simulink model "MotorControlSim_OpenLoopPWM"  (R2025b)
settings: Solver=FixedStepAuto  FixedStep=1e-6
libraries: slpidlib x2, simulink x1
(part 1 of 2)
settings Model: Creator=azmib
settings SolverCC: ZeroCrossControl=EnableAll  MaxZcPerStep=100.0
settings SimscapeCC: SimscapeNominalValues="[{\"value\":\"1\",\"unit\":\"A\"},{\"value\":\"1\",\"unit\":\"bar\"},{\"value\":\"1\",\"unit\":\"cm^2\"},{\"value\":\"1\",\"unit\":\"cm^3/s\"},{\"value\":\"1\",\"unit\":\"kJ/kg\"},{\"value\":\"1\",\"unit\":\"kW\"},{\"value\":\"1\",\"unit\":\"l\"},{\"value\":\"1\",\"unit\":\"N\"},{\"value\":\"1\",\"unit\":\"N*m\"},{\"value\":\"1\",\"unit\":\"V\"},{\"value\":\"0.001\",\"unit\":\"Wb\"}]"  SimscapeLogType=all  SimscapeLogDataHistory=10000.0

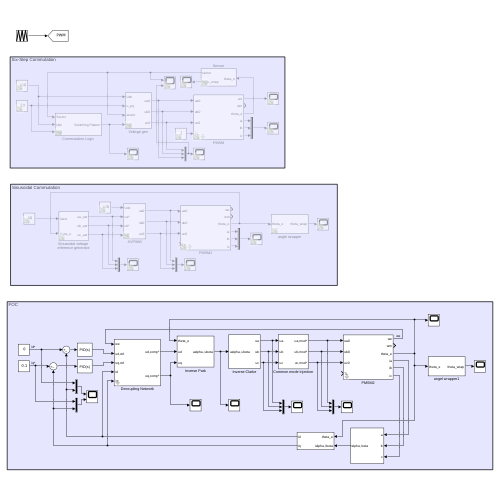
[thumbnail: Simulink's stored preview of the top-level diagram]
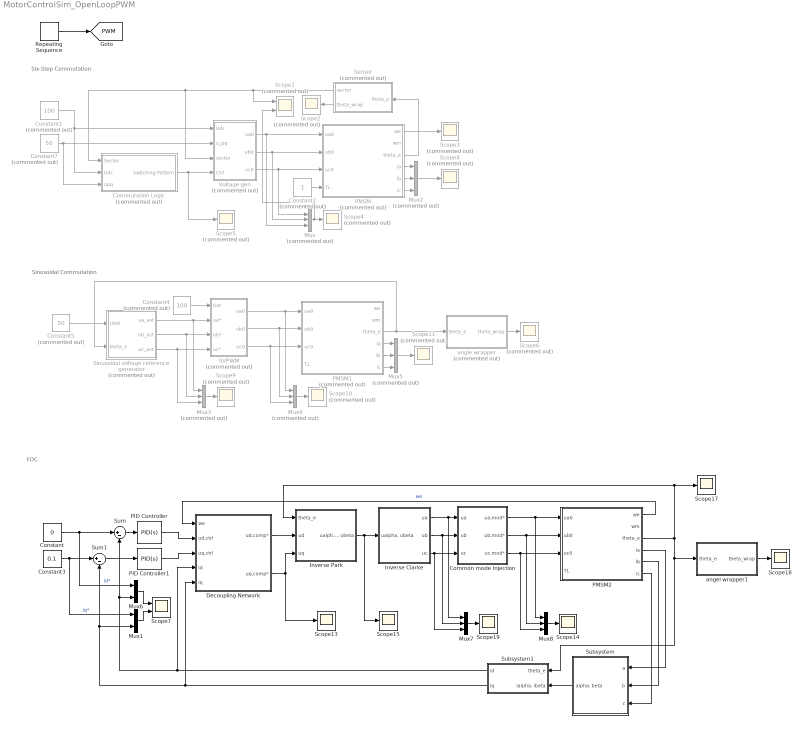
== system MotorControlSim_OpenLoopPWM ==
  note: FOC
  note: Sinusoidal Commutation
  note: Six-Step Commutation
  Common mode Injection : Subsystem
  Commutation Logic : Subsystem  Commented=on
  Constant : Constant  Value=0
  Constant1 : Constant  Commented=on  Value=100
  Constant2 : Constant  Commented=on
  Constant3 : Constant  Value=0.1
  Constant4 : Constant  Commented=on  Value=100
  Constant5 : Constant  Commented=on  Value=50
  Constant7 : Constant  Commented=on  Value=50
  Decoupling Network : Subsystem  mask{Ls=0.002, psi_PM=0.018}
      mask prompts: Ls "pq Inductance"; psi_PM "Permanent magnet flux"
  Inverse Clarke : Subsystem
  Inverse Park : Subsystem
  Mux{,2..5} (5 alike) : Mux  Commented=on  Inputs=3
  Mux1 : Mux  Inputs=2
  Mux6 : Mux  Inputs=2
  Mux7 : Mux  Inputs=3
  Mux8 : Mux  Inputs=3
  PID Controller : slpidlib/PID Controller  Controller=PID  Form=Parallel  TimeDomain=Continuous-time  UseExternalTs=off  SampleTime=-1  IntegratorMethod=Forward Euler  FilterMethod=Forward Euler  ControllerParametersSource=internal  P=15  I=250  UseKiTs=off  D=0  UseExternalDerivativeSource=off  N=100  UseFilter=on  TunerSelectOption=Transfer Function Based (PID Tuner App)  InitialConditionSource=internal  InitialConditionForIntegrator=0  InitialConditionForFilter=0  DifferentiatorICPrevScaledInput=0  ExternalReset=none  TrackingMode=off  Kt=1  LimitOutput=off  SatLimitsSource=internal  UpperSaturationLimit=inf  LowerSaturationLimit=-inf  LinearizeAsGain=on  AntiWindupMode=none  Kb=1  LimitIntegrator=off  UpperIntegratorSaturationLimit=inf  LowerIntegratorSaturationLimit=-inf  POutMin=[]  POutMax=[]  IOutMin=[]  IOutMax=[]  DOutMin=[]  DOutMax=[]  NOutMin=[]  NOutMax=[]  SumOutMin=[]  SumOutMax=[]  SaturationOutMin=[]  SaturationOutMax=[]  PParamMin=[]  PParamMax=[]  IParamMin=[]  IParamMax=[]  DParamMin=[]  DParamMax=[]  NParamMin=[]  NParamMax=[]  KbParamMin=[]  KbParamMax=[]  KtParamMin=[]  KtParamMax=[]  KbOutMin=[]  KbOutMax=[]  KtOutMin=[]  KtOutMax=[]  IntegratorOutMin=[]  IntegratorOutMax=[]  FilterOutMin=[]  FilterOutMax=[]  SumI1OutMin=[]  SumI1OutMax=[]  SumI2OutMin=[]  SumI2OutMax=[]  SumI3OutMin=[]  SumI3OutMax=[]  SumI4OutMin=[]  SumI4OutMax=[]  SumDOutMin=[]  SumDOutMax=[]  DifferentiatorOutMin=[]  DifferentiatorOutMax=[]  FilterDiffOutCoefMin=[]  FilterDiffOutCoefMax=[]  ReciprocalOutMin=[]  ReciprocalOutMax=[]  SumDenOutMin=[]  SumDenOutMax=[]  SumNumOutMin=[]  SumNumOutMax=[]  DivideOutMin=[]  DivideOutMax=[]  UdiffTsProdOutMin=[]  UdiffTsProdOutMax=[]  NTsProdOutMin=[]  NTsProdOutMax=[]  UintegralTsProdOutMin=[]  UintegralTsProdOutMax=[]  UngainTsProdOutMin=[]  UngainTsProdOutMax=[]  ClampingZeroOutDataTypeStr=Inherit: Inherit via back propagation  ClampingZeroOutMin=[]  ClampingZeroOutMax=[]  FilterDenConstantOutDataTypeStr=Inherit: Inherit via back propagation  FilterDenConstantOutMin=[]  FilterDenConstantOutMax=[]  PCopyOutDataTypeStr=Inherit: Inherit via back propagation  PCopyOutMin=[]  PCopyOutMax=[]  NCopyOutDataTypeStr=Inherit: Inherit via back propagation  NCopyOutMin=[]  NCopyOutMax=[]  IntegratorContinuousStateAttributes=''  IntegratorStateMustResolveToSignalObject=off  IntegratorRTWStateStorageClass=Auto  FilterContinuousStateAttributes=''  FilterStateMustResolveToSignalObject=off  FilterRTWStateStorageClass=Auto  ParallelPVariant=InternalParameters  IdealPVariant=Disabled  IVariant=InternalParameters  DVariant=InternalParameters  IntegratorVariant=Continuous  SatVariant=Disabled  AWVariant=Passthrough  PCopyVariant=Disabled  TRVariant=Disabled  FdbkBlocksVariant=Forward  IdealPFdbkVariant=Disabled  SatFdbkVariant=Disabled  DerivativeFilterVariant=ContFilter  NVariant=InternalParameters  NCopyVariant=Disabled  FilterICVariant=InternalICsFilter  IntegratorICVariant=InternalICs  ExternalResetVariant=Disabled  TRSumVariant=Passthrough  SumFdbkVariant=Disabled  SumVariant=Sum_PID  TsampFilterVariant=InternalTs  TsampNgainVariant=Passthrough  TsampIntegralVariant=Disabled_SignalSpec  ExternalSaturationOutDataTypeStr=Inherit: Same as second input  DerivativeSourceVariant=ErrorSignal  PreIntVariant=InternalPreInt
  PID Controller1 : slpidlib/PID Controller  Controller=PID  Form=Parallel  TimeDomain=Continuous-time  UseExternalTs=off  SampleTime=-1  IntegratorMethod=Forward Euler  FilterMethod=Forward Euler  ControllerParametersSource=internal  P=15  I=250  UseKiTs=off  D=0  UseExternalDerivativeSource=off  N=100  UseFilter=on  TunerSelectOption=Transfer Function Based (PID Tuner App)  InitialConditionSource=internal  InitialConditionForIntegrator=0  InitialConditionForFilter=0  DifferentiatorICPrevScaledInput=0  ExternalReset=none  TrackingMode=off  Kt=1  LimitOutput=off  SatLimitsSource=internal  UpperSaturationLimit=inf  LowerSaturationLimit=-inf  LinearizeAsGain=on  AntiWindupMode=none  Kb=1  LimitIntegrator=off  UpperIntegratorSaturationLimit=inf  LowerIntegratorSaturationLimit=-inf  POutMin=[]  POutMax=[]  IOutMin=[]  IOutMax=[]  DOutMin=[]  DOutMax=[]  NOutMin=[]  NOutMax=[]  SumOutMin=[]  SumOutMax=[]  SaturationOutMin=[]  SaturationOutMax=[]  PParamMin=[]  PParamMax=[]  IParamMin=[]  IParamMax=[]  DParamMin=[]  DParamMax=[]  NParamMin=[]  NParamMax=[]  KbParamMin=[]  KbParamMax=[]  KtParamMin=[]  KtParamMax=[]  KbOutMin=[]  KbOutMax=[]  KtOutMin=[]  KtOutMax=[]  IntegratorOutMin=[]  IntegratorOutMax=[]  FilterOutMin=[]  FilterOutMax=[]  SumI1OutMin=[]  SumI1OutMax=[]  SumI2OutMin=[]  SumI2OutMax=[]  SumI3OutMin=[]  SumI3OutMax=[]  SumI4OutMin=[]  SumI4OutMax=[]  SumDOutMin=[]  SumDOutMax=[]  DifferentiatorOutMin=[]  DifferentiatorOutMax=[]  FilterDiffOutCoefMin=[]  FilterDiffOutCoefMax=[]  ReciprocalOutMin=[]  ReciprocalOutMax=[]  SumDenOutMin=[]  SumDenOutMax=[]  SumNumOutMin=[]  SumNumOutMax=[]  DivideOutMin=[]  DivideOutMax=[]  UdiffTsProdOutMin=[]  UdiffTsProdOutMax=[]  NTsProdOutMin=[]  NTsProdOutMax=[]  UintegralTsProdOutMin=[]  UintegralTsProdOutMax=[]  UngainTsProdOutMin=[]  UngainTsProdOutMax=[]  ClampingZeroOutDataTypeStr=Inherit: Inherit via back propagation  ClampingZeroOutMin=[]  ClampingZeroOutMax=[]  FilterDenConstantOutDataTypeStr=Inherit: Inherit via back propagation  FilterDenConstantOutMin=[]  FilterDenConstantOutMax=[]  PCopyOutDataTypeStr=Inherit: Inherit via back propagation  PCopyOutMin=[]  PCopyOutMax=[]  NCopyOutDataTypeStr=Inherit: Inherit via back propagation  NCopyOutMin=[]  NCopyOutMax=[]  IntegratorContinuousStateAttributes=''  IntegratorStateMustResolveToSignalObject=off  IntegratorRTWStateStorageClass=Auto  FilterContinuousStateAttributes=''  FilterStateMustResolveToSignalObject=off  FilterRTWStateStorageClass=Auto  ParallelPVariant=InternalParameters  IdealPVariant=Disabled  IVariant=InternalParameters  DVariant=InternalParameters  IntegratorVariant=Continuous  SatVariant=Disabled  AWVariant=Passthrough  PCopyVariant=Disabled  TRVariant=Disabled  FdbkBlocksVariant=Forward  IdealPFdbkVariant=Disabled  SatFdbkVariant=Disabled  DerivativeFilterVariant=ContFilter  NVariant=InternalParameters  NCopyVariant=Disabled  FilterICVariant=InternalICsFilter  IntegratorICVariant=InternalICs  ExternalResetVariant=Disabled  TRSumVariant=Passthrough  SumFdbkVariant=Disabled  SumVariant=Sum_PID  TsampFilterVariant=InternalTs  TsampNgainVariant=Passthrough  TsampIntegralVariant=Disabled_SignalSpec  ExternalSaturationOutDataTypeStr=Inherit: Same as second input  DerivativeSourceVariant=ErrorSignal  PreIntVariant=InternalPreInt
  PMSM : Subsystem  Commented=on  mask(PMSM){Rs=0.045, Ls=0.002, psi_PM=0.018, p=14, J=2.5e-4, B=1e-3}
      mask prompts: Rs "Phase resistance [Rs]"; Ls "Direct- and  quadrature-axis inductances [Ls]"; psi_PM "Permanent magnet flux linkage [psi_PM]"; p "Pole pairs [p}"; J "Moment of inertia [J]"; B "viscous friction coefficient [B]"
      mask help: Mathematical model of a non-salient permanent magnet synchronous motor (PMSM).
  PMSM1 : Subsystem  Commented=on  mask(PMSM){Rs=0.045, Ls=0.002, psi_PM=0.018, p=14, J=2.5e-4, B=1e-3}
      mask prompts: Rs "Phase resistance [Rs]"; Ls "Direct- and  quadrature-axis inductances [Ls]"; psi_PM "Permanent magnet flux linkage [psi_PM]"; p "Pole pairs [p}"; J "Moment of inertia [J]"; B "viscous friction coefficient [B]"
      mask help: Mathematical model of a non-salient permanent magnet synchronous motor (PMSM).
  PMSM2 : Subsystem  mask(PMSM){Rs=0.045, Ls=0.002, psi_PM=0.018, p=14, J=2.5e-4, B=1e-3}
      mask prompts: Rs "Phase resistance [Rs]"; Ls "Direct- and  quadrature-axis inductances [Ls]"; psi_PM "Permanent magnet flux linkage [psi_PM]"; p "Pole pairs [p}"; J "Moment of inertia [J]"; B "viscous friction coefficient [B]"
      mask help: Mathematical model of a non-salient permanent magnet synchronous motor (PMSM).
  Repeating Sequence : simulink/Sources/Repeating Sequence  rep_seq_t=[0 0.00005 0.0001]  rep_seq_y=[0 1 0]
  SVPWM : Subsystem  Commented=on
  Scope1 : Scope  Commented=on  NumInputPorts=2
      settings: ActiveDisplayYMinimum=0.54492848630705648  ActiveDisplayYMaximum=6.21386272666987
  Scope{2..6,8..11} (9 alike) : Scope  Commented=on
      Scope10 settings: ActiveDisplayYMinimum=-12.499999999999996  ActiveDisplayYMaximum=112.5  DataLoggingVariableName=ScopeData10
      Scope11 settings: ActiveDisplayYMinimum=-61.952484857839465  ActiveDisplayYMaximum=66.897862739349023  DataLoggingVariableName=ScopeData11
      Scope2 settings: ActiveDisplayYMinimum=-44.997868385096346  ActiveDisplayYMaximum=404.99935148550094  DataLoggingVariableName=ScopeData2
      Scope3 settings: ActiveDisplayYMinimum=-84.895577173636241  ActiveDisplayYMaximum=93.106926628518693  DataLoggingVariableName=ScopeData3
      Scope4 settings: ActiveDisplayYMinimum=-12.499999999999996  ActiveDisplayYMaximum=112.5  DataLoggingVariableName=ScopeData4
      Scope5 settings: ActiveDisplayYMinimum=-0.14423076923076919  ActiveDisplayYMaximum=1.1057692307692308  DataLoggingVariableName=ScopeData5
      Scope6 settings: ActiveDisplayYMinimum=-556.861480878076  ActiveDisplayYMaximum=474.54651207001933  DataLoggingVariableName=ScopeData7
      Scope8 settings: ActiveDisplayYMinimum=-802.69476139838889  ActiveDisplayYMaximum=793.38425332468114  DataLoggingVariableName=ScopeData6
      Scope9 settings: ActiveDisplayYMinimum=-126.15384615374161  ActiveDisplayYMaximum=123.84615384570814  DataLoggingVariableName=ScopeData9
  Scope{13..15,17..19} (6 alike) : Scope
      Scope13 settings: ActiveDisplayYMinimum=-1.1385144753965966  ActiveDisplayYMaximum=7.7284276585384992  DataLoggingVariableName=ScopeData16
      Scope14 settings: ActiveDisplayYMinimum=-10.316497807088153  ActiveDisplayYMaximum=10.316497807088153  DataLoggingVariableName=ScopeData14
      Scope15 settings: ActiveDisplayYMinimum=-8.4790995533838753  ActiveDisplayYMaximum=8.4863578557596355  DataLoggingVariableName=ScopeData20
      Scope17 settings: ActiveDisplayYMinimum=-1061.0441841261031  ActiveDisplayYMaximum=9549.39765713493  DataLoggingVariableName=ScopeData17
      Scope18 settings: ActiveDisplayYMinimum=-449.98370924834887  ActiveDisplayYMaximum=449.99720138987811  DataLoggingVariableName=ScopeData18
      Scope19 settings: ActiveDisplayYMinimum=-11.80274291560826  ActiveDisplayYMaximum=11.802630733499404  DataLoggingVariableName=ScopeData19
  Scope7 : Scope  NumInputPorts=2
      settings: ActiveDisplayYMinimum=-5.6255188907389564E-5  ActiveDisplayYMaximum=0.0005062967001665062  DataLoggingVariableName=ScopeData13
  Sensor : Subsystem  Commented=on
  Sinusoidal voltage reference generator : Subsystem  Commented=on
  Subsystem : Subsystem
  Subsystem1 : Subsystem
  Sum : Sum  Inputs=|+-
  Sum1 : Sum  Inputs=|+-
  Voltage gen : Subsystem  Commented=on
  angel wrapper1 : Subsystem
  angle wrapper : Subsystem  Commented=on
  tag scope: PWM=global
  wires:
  Constant2/1 -> PMSM/4(TL)
  Sensor/1(sector) -> Voltage gen/3(sector), Commutation Logic/1(Sector), Scope1/1
  Commutation Logic/1(Switching Pattern) -> Scope5/1, Voltage gen/4(Ctrl)
  Voltage gen/2(ub0) -> Mux/2, PMSM/2(ub0)
  Voltage gen/1(ua0) -> Mux/3, PMSM/1(ua0)
  Voltage gen/3(uc0) -> Mux/1, PMSM/3(uc0)
  PMSM/3(theta_e) -> Sensor/1(theta_e)
  Sensor/2(theta_wrap) -> Scope2/1
  PMSM/1(we) -> Scope3/1
  Mux/1 -> Scope1/2, Scope4/1
  PMSM/5(ib) -> Mux2/2
  PMSM/4(ia) -> Mux2/1
  PMSM/6(ic) -> Mux2/3
  Mux2/1 -> Scope8/1
  PMSM1/3(theta_e) -> Sinusoidal voltage reference generator/2(theta_e), angle wrapper/1(theta_e)
  Sinusoidal voltage reference generator/1(ua_ast) -> Mux3/1, SVPWM/2(ua*)
  Sinusoidal voltage reference generator/2(ub_ast) -> Mux3/2, SVPWM/3(ub*)
  Sinusoidal voltage reference generator/3(uc_ast) -> Mux3/3, SVPWM/4(uc*)
  Mux3/1 -> Scope9/1
  SVPWM/1(ua0) -> PMSM1/1(ua0), Mux4/1
  SVPWM/2(ub0) -> PMSM1/2(ub0), Mux4/2
  SVPWM/3(uc0) -> PMSM1/3(uc0), Mux4/3
  Mux4/1 -> Scope10/1
  PMSM1/4(ia) -> Mux5/1
  PMSM1/5(ib) -> Mux5/2
  Mux5/1 -> Scope11/1
  PMSM1/6(ic) -> Mux5/3
  angle wrapper/1(theta_wrap) -> Scope6/1
  Mux7/1 -> Scope19/1
  Mux8/1 -> Scope14/1
  Inverse Clarke/2(ub) -> Mux7/2, Common mode Injection/2(ub)
  Inverse Clarke/1(ua) -> Mux7/1, Common mode Injection/1(ua)
  PMSM2/6(ic) -> Subsystem/3(c)
  PMSM2/3(theta_e) -> Subsystem1/1(theta_e), angel wrapper1/1(theta_e), Inverse Park/1(theta_e), Scope17/1
  angel wrapper1/1(theta_wrap) -> Scope18/1
  PMSM2/5(ib) -> Subsystem/2(b)
  PMSM2/4(ia) -> Subsystem/1(a)
  Inverse Clarke/3(uc) -> Mux7/3, Common mode Injection/3(uc)
  Inverse Park/1("ualpha, ubeta") -> Scope15/1, Inverse Clarke/1("ualpha, ubeta")
  Constant/1 -> Sum/1, Mux6/1  "id*"
  Constant3/1 -> Sum1/1, Mux1/1  "iq*"
  Decoupling Network/2(uq,comp*) -> Scope13/1, Inverse Park/3(uq)
  Decoupling Network/1(ud,comp*) -> Inverse Park/2(ud)
  PMSM2/1(we) -> Decoupling Network/1(we)  "we"
  Constant4/1 -> SVPWM/1(Udc)
  Constant5/1 -> Sinusoidal voltage reference generator/1(Uast)
  Mux1/1 -> Scope7/2
  Mux6/1 -> Scope7/1
  Constant1/1 -> Commutation Logic/2(Udc), Voltage gen/1(Udc)
  Constant7/1 -> Commutation Logic/3(upq), Voltage gen/2(u_pq)
  Common mode Injection/1(ua,mod*) -> Mux8/1, PMSM2/1(ua0)
  Common mode Injection/2(ub,mod*) -> Mux8/2, PMSM2/2(ub0)
  Common mode Injection/3(uc,mod*) -> Mux8/3, PMSM2/3(uc0)
  Repeating Sequence/1 -> [PWM]
  Subsystem/1("alpha, beta") -> Subsystem1/2("ialpha, ibeta")
  Subsystem1/1(id) -> Sum/2, Mux6/2, Decoupling Network/4(id)
  Subsystem1/2(iq) -> Sum1/2, Mux1/2, Decoupling Network/5(iq)
  Sum/1 -> PID Controller/1
  Sum1/1 -> PID Controller1/1
  PID Controller/1 -> Decoupling Network/2(ud,ctrl)
  PID Controller1/1 -> Decoupling Network/3(uq,ctrl)

== system MotorControlSim_OpenLoopPWM/Common mode Injection ==
  ua : Inport
  ub : Inport  Port=2
  uc : Inport  Port=3
  Add{,2..4} (4 alike) : Sum
  Gain : Gain  Gain=-1/2
  Max : MinMax  Function=max  Inputs=3
  Min : MinMax  Inputs=3
  ua,mod* : Outport
  ub,mod* : Outport  Port=2
  uc,mod* : Outport  Port=3
  wires:
  Add2/1 -> ua,mod*/1  "ua,mod*"
  Add3/1 -> ub,mod*/1  "ub,mod*"
  Min/1 -> Add/2
  Add4/1 -> uc,mod*/1  "uc,mod*"
  Add/1 -> Gain/1
  Gain/1 -> Add2/2, Add3/2, Add4/2  "u0"
  ub/1 -> Max/2, Min/2, Add3/1
  Max/1 -> Add/1
  uc/1 -> Max/3, Min/3, Add4/1
  ua/1 -> Min/1, Max/1, Add2/1

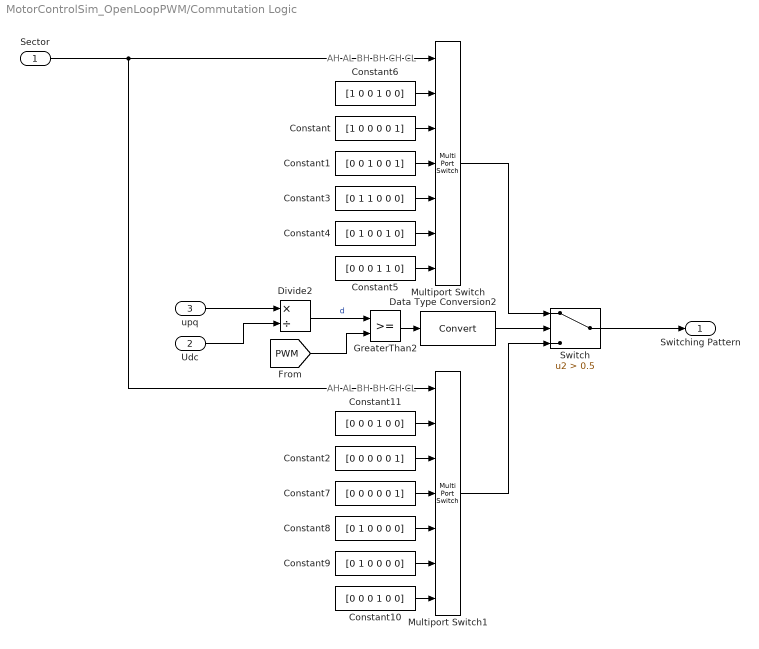
== system MotorControlSim_OpenLoopPWM/Commutation Logic ==
  note: AH AL BH BH CH CL
  note: AH AL BH BH CH CL
  Sector : Inport
  Udc : Inport  Port=2
  upq : Inport  Port=3
  Constant : Constant  Value=[1 0 0 0 0 1]
  Constant1 : Constant  Value=[0 0 1 0 0 1]
  Constant10 : Constant  Value=[0 0 0 1 0 0]
  Constant11 : Constant  Value=[0 0 0 1 0 0]
  Constant2 : Constant  Value=[0 0 0 0 0 1]
  Constant3 : Constant  Value=[0 1 1 0 0 0]
  Constant4 : Constant  Value=[0 1 0 0 1 0]
  Constant5 : Constant  Value=[0 0 0 1 1 0]
  Constant6 : Constant  Value=[1 0 0 1 0 0]
  Constant7 : Constant  Value=[0 0 0 0 0 1]
  Constant8 : Constant  Value=[0 1 0 0 0 0]
  Constant9 : Constant  Value=[0 1 0 0 0 0]
  Data Type Conversion2 : DataTypeConversion  SaturateOnIntegerOverflow=off  RndMeth=Floor
  Divide2 : Product  Inputs=*/
  GreaterThan2 : RelationalOperator  OutDataTypeStr=boolean  RndMeth=Simplest  InputSameDT=off
  Multiport Switch : MultiPortSwitch  Inputs=6  DiagnosticForDefault=None  SaturateOnIntegerOverflow=off  InputSameDT=off
  Multiport Switch1 : MultiPortSwitch  Inputs=6  DiagnosticForDefault=None  SaturateOnIntegerOverflow=off  InputSameDT=off
  Switch : Switch  Criteria=u2 > Threshold  Threshold=0.5  SaturateOnIntegerOverflow=off  InputSameDT=off
  Switching Pattern : Outport
  wires:
  Sector/1 -> Multiport Switch/1, Multiport Switch1/1
  Multiport Switch/1 -> Switch/1
  Multiport Switch1/1 -> Switch/3
  Switch/1 -> Switching Pattern/1
  Constant6/1 -> Multiport Switch/2
  Constant/1 -> Multiport Switch/3
  Constant1/1 -> Multiport Switch/4
  Constant3/1 -> Multiport Switch/5
  Constant5/1 -> Multiport Switch/7
  Constant4/1 -> Multiport Switch/6
  Constant11/1 -> Multiport Switch1/2
  Constant2/1 -> Multiport Switch1/3
  Constant7/1 -> Multiport Switch1/4
  Constant9/1 -> Multiport Switch1/6
  Constant10/1 -> Multiport Switch1/7
  Constant8/1 -> Multiport Switch1/5
  Udc/1 -> Divide2/2
  upq/1 -> Divide2/1
  [PWM] -> GreaterThan2/2
  GreaterThan2/1 -> Data Type Conversion2/1
  Divide2/1 -> GreaterThan2/1  "d"
  Data Type Conversion2/1 -> Switch/2

== system MotorControlSim_OpenLoopPWM/Decoupling Network ==
  we : Inport
  ud,ctrl : Inport  Port=2
  uq,ctrl : Inport  Port=3
  id : Inport  Port=4
  iq : Inport  Port=5
  Add : Sum
  Add4 : Sum  Inputs=+-
  Add5 : Sum
  Constant4 : Constant  Value=psi_PM
  Gain1 : Gain  Gain=Ls
  Gain2 : Gain  Gain=Ls
  Product : Product
  Product1 : Product
  ud,comp* : Outport
  uq,comp* : Outport  Port=2
  wires:
  iq/1 -> Product/1
  Product1/1 -> Add4/2
  Add5/1 -> Product1/2
  Constant4/1 -> Add5/2
  Gain2/1 -> Add5/1
  Add4/1 -> uq,comp*/1  "ud,comp*"
  Product/1 -> Gain1/1
  Gain1/1 -> Add/2
  ud,ctrl/1 -> Add/1
  id/1 -> Gain2/1
  Add/1 -> ud,comp*/1  "ud,comp*"
  we/1 -> Product1/1, Product/2
  uq,ctrl/1 -> Add4/1

== system MotorControlSim_OpenLoopPWM/Inverse Clarke ==
  "ualpha, ubeta" : Inport
  Constant1 : Constant  Value=[1 0; -1/2 sqrt(3)/2; -1/2 -sqrt(3)/2]
  Demux1 : Demux  Outputs=3
  Matrix Multiply : Product  Multiplication=Matrix(*)
  ua : Outport
  ub : Outport  Port=2
  uc : Outport  Port=3
  wires:
  Matrix Multiply/1 -> Demux1/1
  Constant1/1 -> Matrix Multiply/1
  Demux1/2 -> ub/1
  Demux1/3 -> uc/1
  Demux1/1 -> ua/1
  "ualpha, ubeta"/1 -> Matrix Multiply/2

== system MotorControlSim_OpenLoopPWM/Inverse Park ==
  theta_e : Inport
  ud : Inport  Port=2
  uq : Inport  Port=3
  Cos : Trigonometry  Operator=cos
  Gain3 : Gain  Gain=-1
  Matrix Concatenate3 : Concatenate  Mode=Multidimensional array  ConcatenateDimension=2
  Matrix Concatenate4 : Concatenate  Mode=Multidimensional array  ConcatenateDimension=2
  Matrix Concatenate5 : Concatenate  Mode=Multidimensional array
  Mux1 : Mux  Inputs=2
  Product2 : Product  Multiplication=Matrix(*)
  Sin2 : Trigonometry
  "ualpha, ubeta" : Outport
  wires:
  theta_e/1 -> Sin2/1, Cos/1
  Gain3/1 -> Matrix Concatenate3/2
  Cos/1 -> Matrix Concatenate3/1, Matrix Concatenate4/2
  Mux1/1 -> Product2/2
  uq/1 -> Mux1/2
  Matrix Concatenate4/1 -> Matrix Concatenate5/2
  Matrix Concatenate5/1 -> Product2/1
  Product2/1 -> "ualpha, ubeta"/1
  Sin2/1 -> Matrix Concatenate4/1, Gain3/1
  Matrix Concatenate3/1 -> Matrix Concatenate5/1
  ud/1 -> Mux1/1

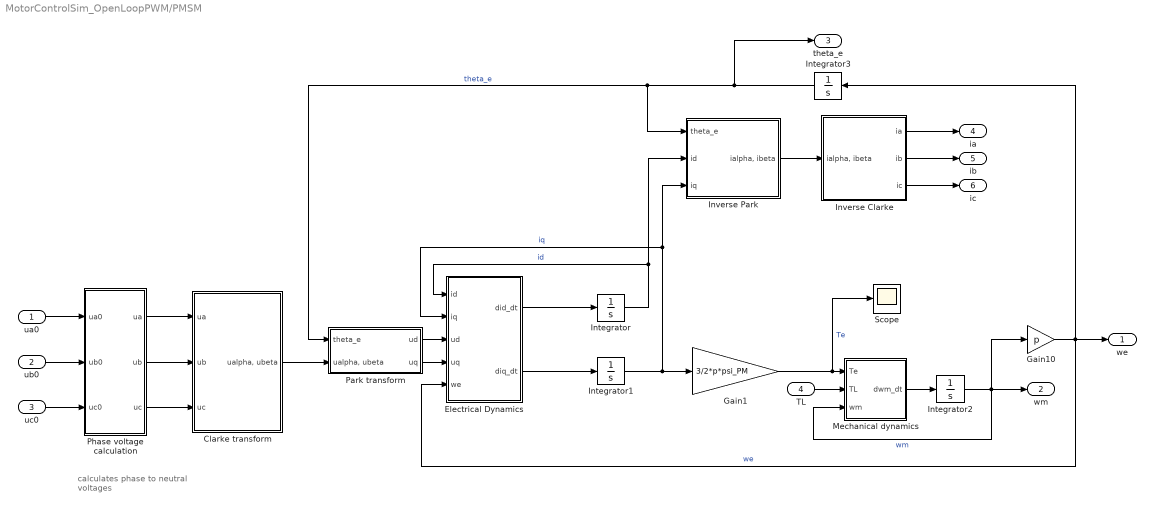
== system MotorControlSim_OpenLoopPWM/PMSM ==
  note: calculates phase to
      | neutral voltages
  ua0 : Inport  Unit=V
  ub0 : Inport  Port=2  Unit=V
  uc0 : Inport  Port=3  Unit=V
  TL : Inport  Port=4
  Clarke transform : Subsystem
  Electrical Dynamics : Subsystem
  Gain1 : Gain  Gain=3/2*p*psi_PM
  Gain10 : Gain  Gain=p
  Integrator{,1..3} (4 alike) : Integrator
  Inverse Clarke : Subsystem
  Inverse Park : Subsystem
  Mechanical dynamics : Subsystem
  Park transform : Subsystem
  Phase voltage calculation : Subsystem
  Scope : Scope
      settings: ActiveDisplayYMinimum=0.88625844411927557  ActiveDisplayYMaximum=1.0374557261199451
  we : Outport
  wm : Outport  Port=2
  theta_e : Outport  Port=3
  ia : Outport  Port=4
  ib : Outport  Port=5
  ic : Outport  Port=6
  wires:
  Integrator3/1 -> Park transform/1(theta_e), Inverse Park/1(theta_e), theta_e/1  "theta_e"
  Gain10/1 -> Integrator3/1, Electrical Dynamics/5(we), we/1  "we"
  Integrator1/1 -> Electrical Dynamics/2(iq), Inverse Park/3(iq), Gain1/1  "iq"
  Gain1/1 -> Scope/1, Mechanical dynamics/1(Te)  "Te"
  TL/1 -> Mechanical dynamics/2(TL)
  Mechanical dynamics/1(dwm_dt) -> Integrator2/1
  Integrator2/1 -> Mechanical dynamics/3(wm), Gain10/1, wm/1  "wm"
  Integrator/1 -> Electrical Dynamics/1(id), Inverse Park/2(id)  "id"
  Electrical Dynamics/1(did_dt) -> Integrator/1
  Electrical Dynamics/2(diq_dt) -> Integrator1/1
  Inverse Park/1("ialpha, ibeta") -> Inverse Clarke/1("ialpha, ibeta")
  Inverse Clarke/2(ib) -> ib/1
  Inverse Clarke/1(ia) -> ia/1
  Inverse Clarke/3(ic) -> ic/1
  Clarke transform/1("ualpha, ubeta") -> Park transform/2("ualpha, ubeta")
  Park transform/1(ud) -> Electrical Dynamics/3(ud)
  Park transform/2(uq) -> Electrical Dynamics/4(uq)
  ub0/1 -> Phase voltage calculation/2(ub0)
  ua0/1 -> Phase voltage calculation/1(ua0)
  uc0/1 -> Phase voltage calculation/3(uc0)
  Phase voltage calculation/2(ub) -> Clarke transform/2(ub)
  Phase voltage calculation/1(ua) -> Clarke transform/1(ua)
  Phase voltage calculation/3(uc) -> Clarke transform/3(uc)

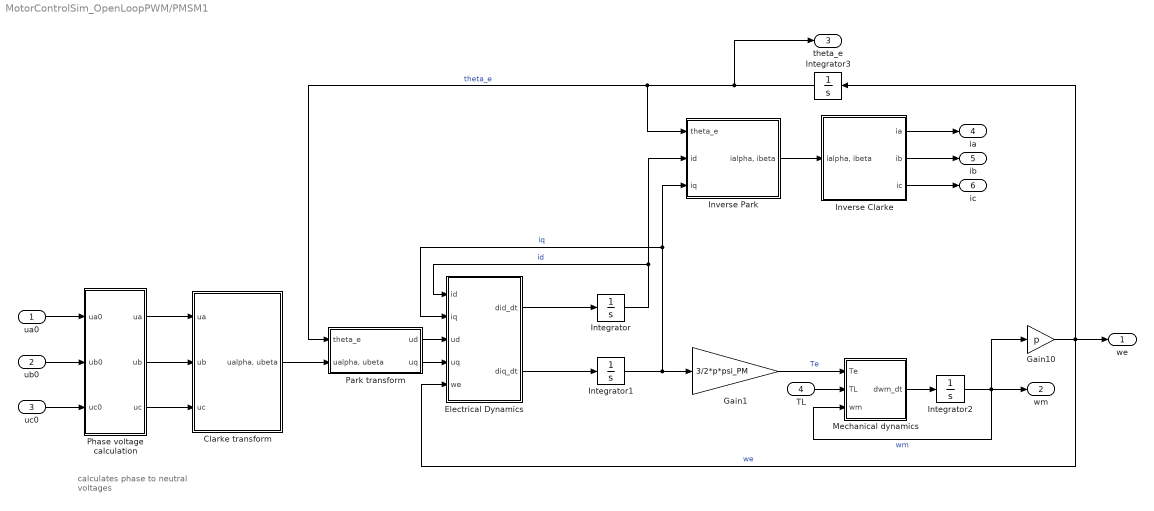
== system MotorControlSim_OpenLoopPWM/PMSM1 ==
  note: calculates phase to
      | neutral voltages
  ua0 : Inport  Unit=V
  ub0 : Inport  Port=2  Unit=V
  uc0 : Inport  Port=3  Unit=V
  TL : Inport  Port=4
  Clarke transform : Subsystem
  Electrical Dynamics : Subsystem
  Gain1 : Gain  Gain=3/2*p*psi_PM
  Gain10 : Gain  Gain=p
  Integrator{,1..3} (4 alike) : Integrator
  Inverse Clarke : Subsystem
  Inverse Park : Subsystem
  Mechanical dynamics : Subsystem
  Park transform : Subsystem
  Phase voltage calculation : Subsystem
  we : Outport
  wm : Outport  Port=2
  theta_e : Outport  Port=3
  ia : Outport  Port=4
  ib : Outport  Port=5
  ic : Outport  Port=6
  wires:
  Integrator3/1 -> Park transform/1(theta_e), Inverse Park/1(theta_e), theta_e/1  "theta_e"
  Gain10/1 -> Integrator3/1, Electrical Dynamics/5(we), we/1  "we"
  Integrator1/1 -> Electrical Dynamics/2(iq), Inverse Park/3(iq), Gain1/1  "iq"
  Gain1/1 -> Mechanical dynamics/1(Te)  "Te"
  TL/1 -> Mechanical dynamics/2(TL)
  Mechanical dynamics/1(dwm_dt) -> Integrator2/1
  Integrator2/1 -> Mechanical dynamics/3(wm), Gain10/1, wm/1  "wm"
  Integrator/1 -> Electrical Dynamics/1(id), Inverse Park/2(id)  "id"
  Electrical Dynamics/1(did_dt) -> Integrator/1
  Electrical Dynamics/2(diq_dt) -> Integrator1/1
  Inverse Park/1("ialpha, ibeta") -> Inverse Clarke/1("ialpha, ibeta")
  Inverse Clarke/2(ib) -> ib/1
  Inverse Clarke/1(ia) -> ia/1
  Inverse Clarke/3(ic) -> ic/1
  Clarke transform/1("ualpha, ubeta") -> Park transform/2("ualpha, ubeta")
  Park transform/1(ud) -> Electrical Dynamics/3(ud)
  Park transform/2(uq) -> Electrical Dynamics/4(uq)
  ub0/1 -> Phase voltage calculation/2(ub0)
  ua0/1 -> Phase voltage calculation/1(ua0)
  uc0/1 -> Phase voltage calculation/3(uc0)
  Phase voltage calculation/2(ub) -> Clarke transform/2(ub)
  Phase voltage calculation/1(ua) -> Clarke transform/1(ua)
  Phase voltage calculation/3(uc) -> Clarke transform/3(uc)

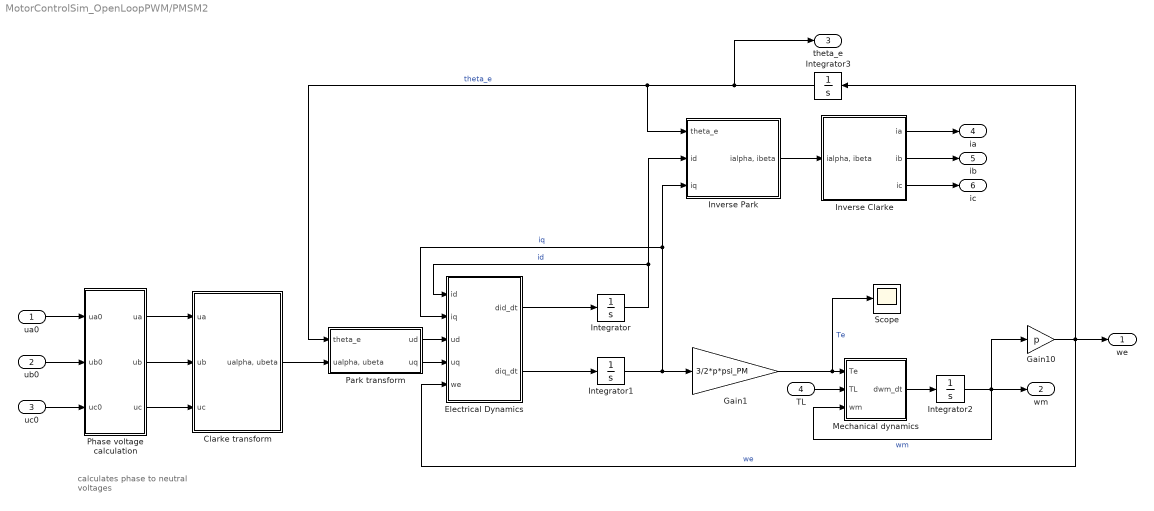
== system MotorControlSim_OpenLoopPWM/PMSM2 ==
  note: calculates phase to
      | neutral voltages
  ua0 : Inport  Unit=V
  ub0 : Inport  Port=2  Unit=V
  uc0 : Inport  Port=3  Unit=V
  TL : Inport  Port=4
  Clarke transform : Subsystem
  Electrical Dynamics : Subsystem
  Gain1 : Gain  Gain=3/2*p*psi_PM
  Gain10 : Gain  Gain=p
  Integrator{,1..3} (4 alike) : Integrator
  Inverse Clarke : Subsystem
  Inverse Park : Subsystem
  Mechanical dynamics : Subsystem
  Park transform : Subsystem
  Phase voltage calculation : Subsystem
  Scope : Scope
      settings: ActiveDisplayYMinimum=0.88625844411927557  ActiveDisplayYMaximum=1.0374557261199451
  we : Outport
  wm : Outport  Port=2
  theta_e : Outport  Port=3
  ia : Outport  Port=4
  ib : Outport  Port=5
  ic : Outport  Port=6
  wires:
  Integrator3/1 -> Park transform/1(theta_e), Inverse Park/1(theta_e), theta_e/1  "theta_e"
  Gain10/1 -> Integrator3/1, Electrical Dynamics/5(we), we/1  "we"
  Integrator1/1 -> Electrical Dynamics/2(iq), Inverse Park/3(iq), Gain1/1  "iq"
  Gain1/1 -> Scope/1, Mechanical dynamics/1(Te)  "Te"
  TL/1 -> Mechanical dynamics/2(TL)
  Mechanical dynamics/1(dwm_dt) -> Integrator2/1
  Integrator2/1 -> Mechanical dynamics/3(wm), Gain10/1, wm/1  "wm"
  Integrator/1 -> Electrical Dynamics/1(id), Inverse Park/2(id)  "id"
  Electrical Dynamics/1(did_dt) -> Integrator/1
  Electrical Dynamics/2(diq_dt) -> Integrator1/1
  Inverse Park/1("ialpha, ibeta") -> Inverse Clarke/1("ialpha, ibeta")
  Inverse Clarke/2(ib) -> ib/1
  Inverse Clarke/1(ia) -> ia/1
  Inverse Clarke/3(ic) -> ic/1
  Clarke transform/1("ualpha, ubeta") -> Park transform/2("ualpha, ubeta")
  Park transform/1(ud) -> Electrical Dynamics/3(ud)
  Park transform/2(uq) -> Electrical Dynamics/4(uq)
  ub0/1 -> Phase voltage calculation/2(ub0)
  ua0/1 -> Phase voltage calculation/1(ua0)
  uc0/1 -> Phase voltage calculation/3(uc0)
  Phase voltage calculation/2(ub) -> Clarke transform/2(ub)
  Phase voltage calculation/1(ua) -> Clarke transform/1(ua)
  Phase voltage calculation/3(uc) -> Clarke transform/3(uc)

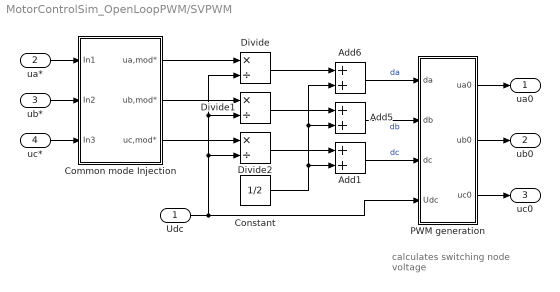
== system MotorControlSim_OpenLoopPWM/SVPWM ==
  note: calculates switching node
      | voltage
  Udc : Inport
  ua* : Inport  Port=2
  ub* : Inport  Port=3
  uc* : Inport  Port=4
  Add1 : Sum
  Add5 : Sum
  Add6 : Sum
  Common mode Injection : Subsystem
  Constant : Constant  Value=1/2
  Divide : Product  Inputs=*/
  Divide1 : Product  Inputs=*/
  Divide2 : Product  Inputs=*/
  PWM generation : Subsystem
  ua0 : Outport
  ub0 : Outport  Port=2
  uc0 : Outport  Port=3
  wires:
  Divide/1 -> Add6/1
  Divide1/1 -> Add5/1
  Divide2/1 -> Add1/1
  Constant/1 -> Add1/2, Add5/2, Add6/2
  Udc/1 -> PWM generation/4(Udc), Divide2/2, Divide1/2, Divide/2
  ua*/1 -> Common mode Injection/1(In1)
  ub*/1 -> Common mode Injection/2(In2)
  uc*/1 -> Common mode Injection/3(In3)
  Common mode Injection/1(ua,mod*) -> Divide/1
  Common mode Injection/2(ub,mod*) -> Divide1/1
  Common mode Injection/3(uc,mod*) -> Divide2/1
  Add6/1 -> PWM generation/1(da)  "da"
  Add5/1 -> PWM generation/2(db)  "db"
  Add1/1 -> PWM generation/3(dc)  "dc"
  PWM generation/1(ua0) -> ua0/1
  PWM generation/2(ub0) -> ub0/1
  PWM generation/3(uc0) -> uc0/1

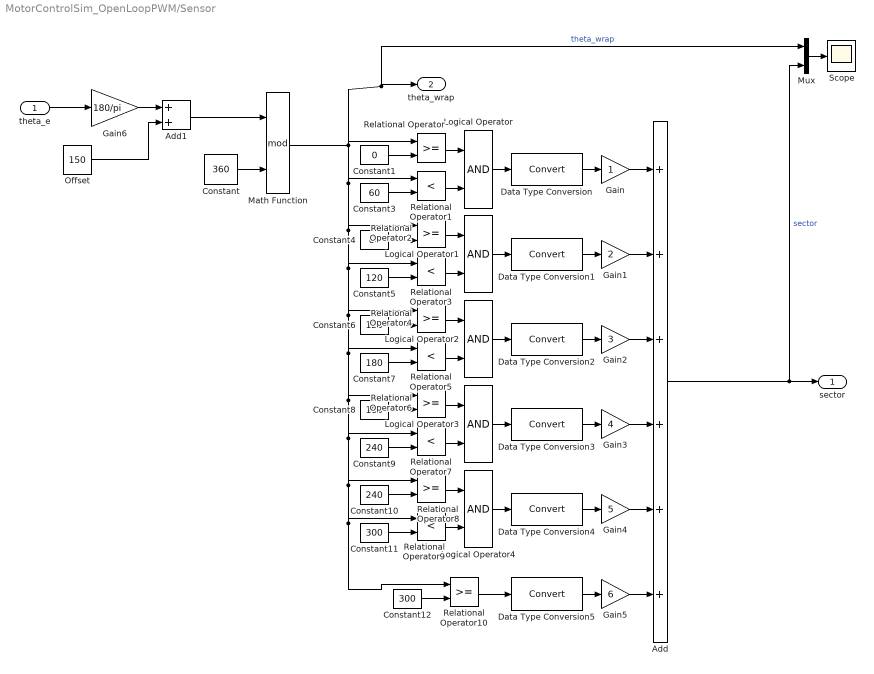
== system MotorControlSim_OpenLoopPWM/Sensor ==
  theta_e : Inport
  Add : Sum  Inputs=++++++
  Add1 : Sum
  Constant : Constant  Value=360
  Constant1 : Constant  Value=0
  Constant10 : Constant  Value=240
  Constant11 : Constant  Value=300
  Constant12 : Constant  Value=300
  Constant3 : Constant  Value=60
  Constant4 : Constant  Value=60
  Constant5 : Constant  Value=120
  Constant6 : Constant  Value=120
  Constant7 : Constant  Value=180
  Constant8 : Constant  Value=180
  Constant9 : Constant  Value=240
  Data Type Conversion{,1..5} (6 alike) : DataTypeConversion  SaturateOnIntegerOverflow=off  RndMeth=Floor
  Gain : Gain
  Gain1 : Gain  Gain=2
  Gain2 : Gain  Gain=3
  Gain3 : Gain  Gain=4
  Gain4 : Gain  Gain=5
  Gain5 : Gain  Gain=6
  Gain6 : Gain  Gain=180/pi
  Logical Operator{,1..4} (5 alike) : Logic  AllPortsSameDT=off  OutDataTypeStr=boolean
  Math Function : Math  Operator=mod
  Mux : Mux  Inputs=2
  Offset : Constant  Value=150
  Relational Operator{,2,4,6,8,10} (6 alike) : RelationalOperator  OutDataTypeStr=boolean  RndMeth=Simplest  InputSameDT=off
  Relational Operator{1,3,5,7,9} (5 alike) : RelationalOperator  Operator=<  OutDataTypeStr=boolean  RndMeth=Simplest  InputSameDT=off
  Scope : Scope
      settings: ActiveDisplayYMinimum=-39.26586921535646  ActiveDisplayYMaximum=393.39282293820821  DataLoggingVariableName=ScopeData8
  sector : Outport
  theta_wrap : Outport  Port=2
  wires:
  Data Type Conversion2/1 -> Gain2/1
  Constant5/1 -> Relational Operator3/2
  Relational Operator6/1 -> Logical Operator3/1
  Gain5/1 -> Add/6
  Gain3/1 -> Add/4
  Data Type Conversion5/1 -> Gain5/1
  Relational Operator7/1 -> Logical Operator3/2
  Gain2/1 -> Add/3
  Constant10/1 -> Relational Operator8/2
  Relational Operator4/1 -> Logical Operator2/1
  Constant/1 -> Math Function/2
  Constant8/1 -> Relational Operator6/2
  Math Function/1 -> Mux/1, theta_wrap/1, Relational Operator/1, Relational Operator2/1, Relational Operator4/1, Relational Operator10/1, Relational Operator9/1, Relational Operator8/1, Relational Operator7/1, Relational Operator6/1, Relational Operator5/1, Relational Operator3/1, Relational Operator1/1  "theta_wrap"
  Constant12/1 -> Relational Operator10/2
  Constant6/1 -> Relational Operator4/2
  Relational Operator2/1 -> Logical Operator1/1
  Logical Operator2/1 -> Data Type Conversion2/1
  Data Type Conversion1/1 -> Gain1/1
  Relational Operator1/1 -> Logical Operator/2
  Constant11/1 -> Relational Operator9/2
  Add/1 -> Mux/2, sector/1  "sector"
  Logical Operator3/1 -> Data Type Conversion3/1
  Relational Operator5/1 -> Logical Operator2/2
  Relational Operator/1 -> Logical Operator/1
  Gain4/1 -> Add/5
  Logical Operator/1 -> Data Type Conversion/1
  Data Type Conversion3/1 -> Gain3/1
  Gain/1 -> Add/1
  Constant7/1 -> Relational Operator5/2
  Constant3/1 -> Relational Operator1/2
  Relational Operator9/1 -> Logical Operator4/2
  Constant9/1 -> Relational Operator7/2
  Constant4/1 -> Relational Operator2/2
  Logical Operator1/1 -> Data Type Conversion1/1
  Data Type Conversion4/1 -> Gain4/1
  Constant1/1 -> Relational Operator/2
  Logical Operator4/1 -> Data Type Conversion4/1
  Data Type Conversion/1 -> Gain/1
  Gain1/1 -> Add/2
  Relational Operator3/1 -> Logical Operator1/2
  Relational Operator8/1 -> Logical Operator4/1
  theta_e/1 -> Gain6/1
  Relational Operator10/1 -> Data Type Conversion5/1
  Gain6/1 -> Add1/1
  Add1/1 -> Math Function/1
  Offset/1 -> Add1/2
  Mux/1 -> Scope/1

== system MotorControlSim_OpenLoopPWM/Sinusoidal voltage reference generator ==
  Uast : Inport
  theta_e : Inport  Port=2
  Constant : Constant  Value=2*pi/3
  Product : Product
  Product1 : Product
  Product2 : Product
  Sin : Trigonometry
  Sin1 : Trigonometry
  Sin2 : Trigonometry
  Sum1 : Sum  Inputs=|+-
  Sum2 : Sum  Inputs=|++
  ua_ast : Outport
  ub_ast : Outport  Port=2
  uc_ast : Outport  Port=3
  wires:
  Sum2/1 -> Sin2/1
  Product/1 -> uc_ast/1  "uc_ast"
  Sin1/1 -> Product1/2
  Constant/1 -> Sum2/2, Sum1/2
  Sum1/1 -> Sin1/1
  theta_e/1 -> Sin/1, Sum1/1, Sum2/1
  Sin2/1 -> Product/2
  Sin/1 -> Product2/2
  Product2/1 -> ua_ast/1  "ua_ast"
  Product1/1 -> ub_ast/1  "ub_ast"
  Uast/1 -> Product2/1, Product1/1, Product/1

== system MotorControlSim_OpenLoopPWM/Subsystem ==
  a : Inport
  b : Inport  Port=2
  c : Inport  Port=3
  Constant : Constant  Value=[1 -1/2 -1/2; 0 sqrt(3)/2 -sqrt(3)/2]
  Gain2 : Gain  Gain=2/3
  Mux : Mux  Inputs=3
  Product : Product  Multiplication=Matrix(*)
  "alpha, beta" : Outport
  wires:
  Gain2/1 -> Product/1
  b/1 -> Mux/2
  Constant/1 -> Gain2/1
  Mux/1 -> Product/2
  Product/1 -> "alpha, beta"/1
  c/1 -> Mux/3
  a/1 -> Mux/1

== system MotorControlSim_OpenLoopPWM/Subsystem1 ==
  theta_e : Inport
  "ialpha, ibeta" : Inport  Port=2
  Demux : Demux  Outputs=2
  Gain : Gain  Gain=-1
  Matrix Concatenate : Concatenate  Mode=Multidimensional array  ConcatenateDimension=2
  Matrix Concatenate1 : Concatenate  Mode=Multidimensional array  ConcatenateDimension=2
  Matrix Concatenate2 : Concatenate  Mode=Multidimensional array
  Product1 : Product  Multiplication=Matrix(*)
  Sin : Trigonometry  Operator=cos
  Sin1 : Trigonometry
  id : Outport
  iq : Outport  Port=2
  wires:
  Demux/2 -> iq/1  "uq"
  Product1/1 -> Demux/1  "ud, uq"
  Gain/1 -> Matrix Concatenate1/1
  Matrix Concatenate1/1 -> Matrix Concatenate2/2
  Sin1/1 -> Gain/1, Matrix Concatenate/2
  Matrix Concatenate2/1 -> Product1/1
  Matrix Concatenate/1 -> Matrix Concatenate2/1
  Sin/1 -> Matrix Concatenate/1, Matrix Concatenate1/2
  theta_e/1 -> Sin1/1, Sin/1
  Demux/1 -> id/1  "ud"
  "ialpha, ibeta"/1 -> Product1/2

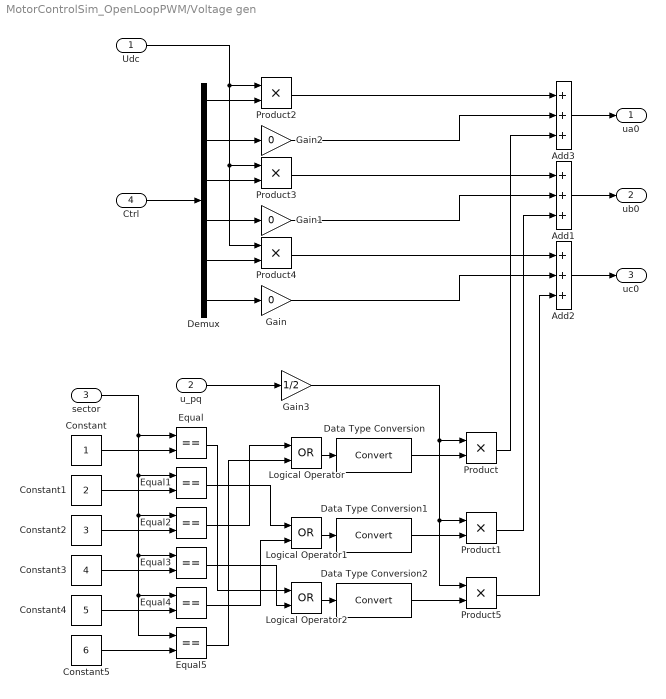
== system MotorControlSim_OpenLoopPWM/Voltage gen ==
  Udc : Inport
  u_pq : Inport  Port=2
  sector : Inport  Port=3
  Ctrl : Inport  Port=4
  Add1 : Sum  Inputs=+++
  Add2 : Sum  Inputs=+++
  Add3 : Sum  Inputs=+++
  Constant : Constant
  Constant1 : Constant  Value=2
  Constant2 : Constant  Value=3
  Constant3 : Constant  Value=4
  Constant4 : Constant  Value=5
  Constant5 : Constant  Value=6
  Data Type Conversion : DataTypeConversion  SaturateOnIntegerOverflow=off  RndMeth=Floor
  Data Type Conversion1 : DataTypeConversion  SaturateOnIntegerOverflow=off  RndMeth=Floor
  Data Type Conversion2 : DataTypeConversion  SaturateOnIntegerOverflow=off  RndMeth=Floor
  Demux : Demux  Outputs=6
  Equal{,1..5} (6 alike) : RelationalOperator  Operator===  OutDataTypeStr=boolean  RndMeth=Simplest  InputSameDT=off
  Gain : Gain  Gain=0
  Gain1 : Gain  Gain=0
  Gain2 : Gain  Gain=0
  Gain3 : Gain  Gain=1/2
  Logical Operator : Logic  Operator=OR  AllPortsSameDT=off  OutDataTypeStr=boolean
  Logical Operator1 : Logic  Operator=OR  AllPortsSameDT=off  OutDataTypeStr=boolean
  Logical Operator2 : Logic  Operator=OR  AllPortsSameDT=off  OutDataTypeStr=boolean
  Product{,1..5} (6 alike) : Product
  ua0 : Outport
  ub0 : Outport  Port=2
  uc0 : Outport  Port=3
  wires:
  Demux/3 -> Product3/2
  Udc/1 -> Product4/1, Product3/1, Product2/1
  Ctrl/1 -> Demux/1
  Demux/1 -> Product2/2
  Demux/5 -> Product4/2
  Product2/1 -> Add3/1
  Demux/6 -> Gain/1
  Demux/4 -> Gain1/1
  Demux/2 -> Gain2/1
  Gain2/1 -> Add3/2
  Data Type Conversion/1 -> Product/2
  Data Type Conversion1/1 -> Product1/2
  Data Type Conversion2/1 -> Product5/2
  Gain3/1 -> Product/1, Product1/1, Product5/1
  Product3/1 -> Add1/1
  Gain1/1 -> Add1/2
  Product4/1 -> Add2/1
  Gain/1 -> Add2/2
  Product/1 -> Add3/3
  Product1/1 -> Add1/3
  Product5/1 -> Add2/3
  Add3/1 -> ua0/1
  Add1/1 -> ub0/1
  Add2/1 -> uc0/1
  sector/1 -> Equal5/1, Equal4/1, Equal3/1, Equal2/1, Equal1/1, Equal/1
  Constant/1 -> Equal/2
  Constant1/1 -> Equal1/2
  Constant2/1 -> Equal2/2
  Constant3/1 -> Equal3/2
  Constant4/1 -> Equal4/2
  Constant5/1 -> Equal5/2
  Logical Operator/1 -> Data Type Conversion/1
  Logical Operator1/1 -> Data Type Conversion1/1
  Logical Operator2/1 -> Data Type Conversion2/1
  Equal2/1 -> Logical Operator/1
  Equal5/1 -> Logical Operator/2
  Equal1/1 -> Logical Operator1/1
  Equal4/1 -> Logical Operator1/2
  Equal3/1 -> Logical Operator2/2
  Equal/1 -> Logical Operator2/1
  u_pq/1 -> Gain3/1

== system MotorControlSim_OpenLoopPWM/angel wrapper1 ==
  theta_e : Inport
  Constant : Constant  Value=360
  Gain6 : Gain  Gain=180/pi
  Math Function : Math  Operator=rem
  theta_wrap : Outport
  wires:
  Constant/1 -> Math Function/2
  Gain6/1 -> Math Function/1  "theta_deg"
  theta_e/1 -> Gain6/1
  Math Function/1 -> theta_wrap/1  "theta_wrap"

== system MotorControlSim_OpenLoopPWM/angle wrapper ==
  theta_e : Inport
  Constant : Constant  Value=360
  Gain6 : Gain  Gain=180/pi
  Math Function : Math  Operator=rem
  theta_wrap : Outport
  wires:
  Constant/1 -> Math Function/2
  Gain6/1 -> Math Function/1  "theta_deg"
  theta_e/1 -> Gain6/1
  Math Function/1 -> theta_wrap/1  "theta_wrap"

== system MotorControlSim_OpenLoopPWM/PMSM/Clarke transform ==
  ua : Inport
  ub : Inport  Port=2
  uc : Inport  Port=3
  Constant : Constant  Value=[1 -1/2 -1/2; 0 sqrt(3)/2 -sqrt(3)/2]
  Gain2 : Gain  Gain=2/3
  Mux : Mux  Inputs=3
  Product : Product  Multiplication=Matrix(*)
  "ualpha, ubeta" : Outport
  wires:
  Gain2/1 -> Product/1
  ub/1 -> Mux/2
  Constant/1 -> Gain2/1
  Mux/1 -> Product/2
  Product/1 -> "ualpha, ubeta"/1
  uc/1 -> Mux/3
  ua/1 -> Mux/1

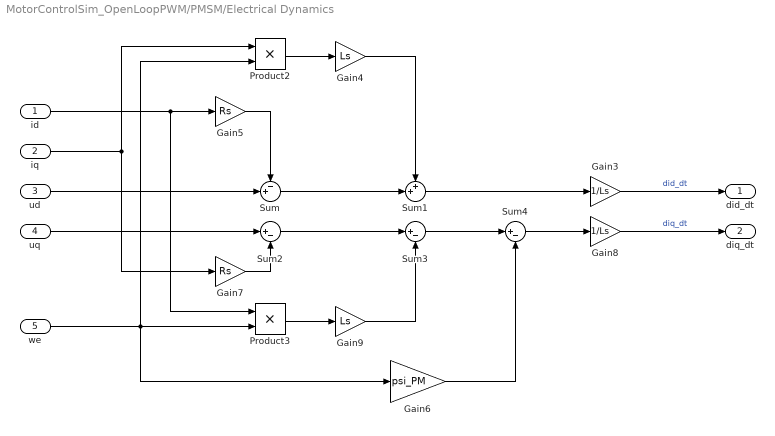
== system MotorControlSim_OpenLoopPWM/PMSM/Electrical Dynamics ==
  id : Inport
  iq : Inport  Port=2
  ud : Inport  Port=3
  uq : Inport  Port=4
  we : Inport  Port=5
  Gain3 : Gain  Gain=1/Ls
  Gain4 : Gain  Gain=Ls
  Gain5 : Gain  Gain=Rs
  Gain6 : Gain  Gain=psi_PM
  Gain7 : Gain  Gain=Rs
  Gain8 : Gain  Gain=1/Ls
  Gain9 : Gain  Gain=Ls
  Product2 : Product
  Product3 : Product
  Sum : Sum  Inputs=-+|
  Sum1 : Sum  Inputs=++|
  Sum2 : Sum  Inputs=|+-
  Sum3 : Sum  Inputs=|+-
  Sum4 : Sum  Inputs=|+-
  did_dt : Outport
  diq_dt : Outport  Port=2
  wires:
  Product2/1 -> Gain4/1
  Gain9/1 -> Sum3/2
  Gain7/1 -> Sum2/2
  Sum/1 -> Sum1/2
  iq/1 -> Gain7/1, Product2/1
  Product3/1 -> Gain9/1
  Sum4/1 -> Gain8/1
  ud/1 -> Sum/2
  Gain4/1 -> Sum1/1
  Gain6/1 -> Sum4/2
  Gain8/1 -> diq_dt/1  "diq_dt"
  Gain5/1 -> Sum/1
  id/1 -> Product3/1, Gain5/1
  uq/1 -> Sum2/1
  we/1 -> Product2/2, Gain6/1, Product3/2
  Sum3/1 -> Sum4/1
  Sum1/1 -> Gain3/1
  Gain3/1 -> did_dt/1  "did_dt"
  Sum2/1 -> Sum3/1

== system MotorControlSim_OpenLoopPWM/PMSM/Inverse Clarke ==
  "ialpha, ibeta" : Inport
  Constant1 : Constant  Value=[1 0; -1/2 sqrt(3)/2; -1/2 -sqrt(3)/2]
  Demux1 : Demux  Outputs=3
  Matrix Multiply : Product  Multiplication=Matrix(*)
  ia : Outport
  ib : Outport  Port=2
  ic : Outport  Port=3
  wires:
  Matrix Multiply/1 -> Demux1/1
  Constant1/1 -> Matrix Multiply/1
  Demux1/2 -> ib/1  "ib"
  Demux1/3 -> ic/1  "ic"
  Demux1/1 -> ia/1  "ia"
  "ialpha, ibeta"/1 -> Matrix Multiply/2

== system MotorControlSim_OpenLoopPWM/PMSM/Inverse Park ==
  theta_e : Inport
  id : Inport  Port=2
  iq : Inport  Port=3
  Cos : Trigonometry  Operator=cos
  Gain3 : Gain  Gain=-1
  Matrix Concatenate3 : Concatenate  Mode=Multidimensional array  ConcatenateDimension=2
  Matrix Concatenate4 : Concatenate  Mode=Multidimensional array  ConcatenateDimension=2
  Matrix Concatenate5 : Concatenate  Mode=Multidimensional array
  Mux1 : Mux  Inputs=2
  Product2 : Product  Multiplication=Matrix(*)
  Sin2 : Trigonometry
  "ialpha, ibeta" : Outport
  wires:
  theta_e/1 -> Sin2/1, Cos/1
  Gain3/1 -> Matrix Concatenate3/2
  Cos/1 -> Matrix Concatenate3/1, Matrix Concatenate4/2
  Mux1/1 -> Product2/2
  iq/1 -> Mux1/2
  Matrix Concatenate4/1 -> Matrix Concatenate5/2
  Matrix Concatenate5/1 -> Product2/1
  Product2/1 -> "ialpha, ibeta"/1  "ialpha, ibeta"
  Sin2/1 -> Matrix Concatenate4/1, Gain3/1
  Matrix Concatenate3/1 -> Matrix Concatenate5/1
  id/1 -> Mux1/1

== system MotorControlSim_OpenLoopPWM/PMSM/Mechanical dynamics ==
  Te : Inport
  TL : Inport  Port=2
  wm : Inport  Port=3
  Gain7 : Gain  Gain=1/J
  Gain9 : Gain  Gain=B
  Sum5 : Sum  Inputs=|+-
  Sum6 : Sum  Inputs=|+-
  dwm_dt : Outport
  wires:
  Gain9/1 -> Sum6/2
  TL/1 -> Sum5/2
  Te/1 -> Sum5/1
  Sum6/1 -> Gain7/1
  wm/1 -> Gain9/1
  Sum5/1 -> Sum6/1
  Gain7/1 -> dwm_dt/1  "dwm_dt"

== system MotorControlSim_OpenLoopPWM/PMSM/Park transform ==
  theta_e : Inport
  "ualpha, ubeta" : Inport  Port=2
  Demux : Demux  Outputs=2
  Gain : Gain  Gain=-1
  Matrix Concatenate : Concatenate  Mode=Multidimensional array  ConcatenateDimension=2
  Matrix Concatenate1 : Concatenate  Mode=Multidimensional array  ConcatenateDimension=2
  Matrix Concatenate2 : Concatenate  Mode=Multidimensional array
  Product1 : Product  Multiplication=Matrix(*)
  Sin : Trigonometry  Operator=cos
  Sin1 : Trigonometry
  ud : Outport
  uq : Outport  Port=2
  wires:
  Demux/2 -> uq/1  "uq"
  Product1/1 -> Demux/1  "ud, uq"
  Gain/1 -> Matrix Concatenate1/1
  Matrix Concatenate1/1 -> Matrix Concatenate2/2
  Sin1/1 -> Gain/1, Matrix Concatenate/2
  Matrix Concatenate2/1 -> Product1/1
  Matrix Concatenate/1 -> Matrix Concatenate2/1
  Sin/1 -> Matrix Concatenate/1, Matrix Concatenate1/2
  theta_e/1 -> Sin1/1, Sin/1
  Demux/1 -> ud/1  "ud"
  "ualpha, ubeta"/1 -> Product1/2

== system MotorControlSim_OpenLoopPWM/PMSM/Phase voltage calculation ==
  ua0 : Inport
  ub0 : Inport  Port=2
  uc0 : Inport  Port=3
  Add : Sum  Inputs=+++
  Gain : Gain  Gain=1/3
  Subtract : Sum  Inputs=+-
  Subtract1 : Sum  Inputs=+-
  Subtract2 : Sum  Inputs=+-
  ua : Outport
  ub : Outport  Port=2
  uc : Outport  Port=3
  wires:
  uc0/1 -> Add/3, Subtract2/1
  Subtract2/1 -> uc/1
  Subtract/1 -> ua/1
  Gain/1 -> Subtract/2, Subtract1/2, Subtract2/2  "un"
  Add/1 -> Gain/1
  ua0/1 -> Subtract/1, Add/1
  ub0/1 -> Add/2, Subtract1/1
  Subtract1/1 -> ub/1

== system MotorControlSim_OpenLoopPWM/PMSM1/Clarke transform ==
  ua : Inport
  ub : Inport  Port=2
  uc : Inport  Port=3
  Constant : Constant  Value=[1 -1/2 -1/2; 0 sqrt(3)/2 -sqrt(3)/2]
  Gain2 : Gain  Gain=2/3
  Mux : Mux  Inputs=3
  Product : Product  Multiplication=Matrix(*)
  "ualpha, ubeta" : Outport
  wires:
  Gain2/1 -> Product/1
  ub/1 -> Mux/2
  Constant/1 -> Gain2/1
  Mux/1 -> Product/2
  Product/1 -> "ualpha, ubeta"/1
  uc/1 -> Mux/3
  ua/1 -> Mux/1

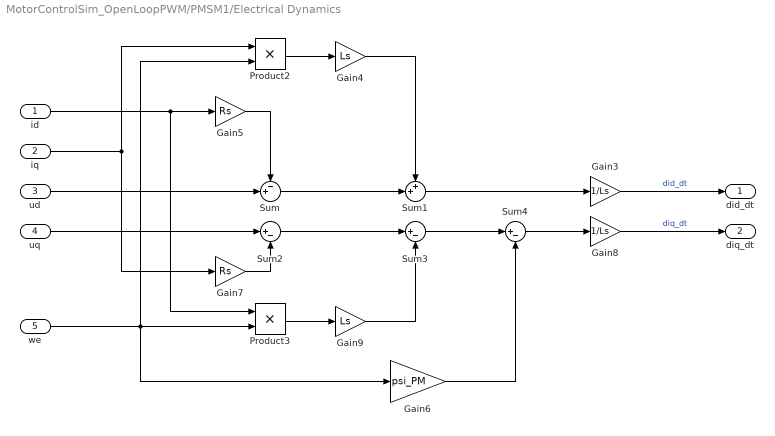
== system MotorControlSim_OpenLoopPWM/PMSM1/Electrical Dynamics ==
  id : Inport
  iq : Inport  Port=2
  ud : Inport  Port=3
  uq : Inport  Port=4
  we : Inport  Port=5
  Gain3 : Gain  Gain=1/Ls
  Gain4 : Gain  Gain=Ls
  Gain5 : Gain  Gain=Rs
  Gain6 : Gain  Gain=psi_PM
  Gain7 : Gain  Gain=Rs
  Gain8 : Gain  Gain=1/Ls
  Gain9 : Gain  Gain=Ls
  Product2 : Product
  Product3 : Product
  Sum : Sum  Inputs=-+|
  Sum1 : Sum  Inputs=++|
  Sum2 : Sum  Inputs=|+-
  Sum3 : Sum  Inputs=|+-
  Sum4 : Sum  Inputs=|+-
  did_dt : Outport
  diq_dt : Outport  Port=2
  wires:
  Product2/1 -> Gain4/1
  Gain9/1 -> Sum3/2
  Gain7/1 -> Sum2/2
  Sum/1 -> Sum1/2
  iq/1 -> Gain7/1, Product2/1
  Product3/1 -> Gain9/1
  Sum4/1 -> Gain8/1
  ud/1 -> Sum/2
  Gain4/1 -> Sum1/1
  Gain6/1 -> Sum4/2
  Gain8/1 -> diq_dt/1  "diq_dt"
  Gain5/1 -> Sum/1
  id/1 -> Product3/1, Gain5/1
  uq/1 -> Sum2/1
  we/1 -> Product2/2, Gain6/1, Product3/2
  Sum3/1 -> Sum4/1
  Sum1/1 -> Gain3/1
  Gain3/1 -> did_dt/1  "did_dt"
  Sum2/1 -> Sum3/1

== system MotorControlSim_OpenLoopPWM/PMSM1/Inverse Clarke ==
  "ialpha, ibeta" : Inport
  Constant1 : Constant  Value=[1 0; -1/2 sqrt(3)/2; -1/2 -sqrt(3)/2]
  Demux1 : Demux  Outputs=3
  Matrix Multiply : Product  Multiplication=Matrix(*)
  ia : Outport
  ib : Outport  Port=2
  ic : Outport  Port=3
  wires:
  Matrix Multiply/1 -> Demux1/1
  Constant1/1 -> Matrix Multiply/1
  Demux1/2 -> ib/1  "ib"
  Demux1/3 -> ic/1  "ic"
  Demux1/1 -> ia/1  "ia"
  "ialpha, ibeta"/1 -> Matrix Multiply/2

== system MotorControlSim_OpenLoopPWM/PMSM1/Inverse Park ==
  theta_e : Inport
  id : Inport  Port=2
  iq : Inport  Port=3
  Cos : Trigonometry  Operator=cos
  Gain3 : Gain  Gain=-1
  Matrix Concatenate3 : Concatenate  Mode=Multidimensional array  ConcatenateDimension=2
  Matrix Concatenate4 : Concatenate  Mode=Multidimensional array  ConcatenateDimension=2
  Matrix Concatenate5 : Concatenate  Mode=Multidimensional array
  Mux1 : Mux  Inputs=2
  Product2 : Product  Multiplication=Matrix(*)
  Sin2 : Trigonometry
  "ialpha, ibeta" : Outport
  wires:
  theta_e/1 -> Sin2/1, Cos/1
  Gain3/1 -> Matrix Concatenate3/2
  Cos/1 -> Matrix Concatenate3/1, Matrix Concatenate4/2
  Mux1/1 -> Product2/2
  iq/1 -> Mux1/2
  Matrix Concatenate4/1 -> Matrix Concatenate5/2
  Matrix Concatenate5/1 -> Product2/1
  Product2/1 -> "ialpha, ibeta"/1  "ialpha, ibeta"
  Sin2/1 -> Matrix Concatenate4/1, Gain3/1
  Matrix Concatenate3/1 -> Matrix Concatenate5/1
  id/1 -> Mux1/1

== system MotorControlSim_OpenLoopPWM/PMSM1/Mechanical dynamics ==
  Te : Inport
  TL : Inport  Port=2
  wm : Inport  Port=3
  Gain7 : Gain  Gain=1/J
  Gain9 : Gain  Gain=B
  Sum5 : Sum  Inputs=|+-
  Sum6 : Sum  Inputs=|+-
  dwm_dt : Outport
  wires:
  Gain9/1 -> Sum6/2
  TL/1 -> Sum5/2
  Te/1 -> Sum5/1
  Sum6/1 -> Gain7/1
  wm/1 -> Gain9/1
  Sum5/1 -> Sum6/1
  Gain7/1 -> dwm_dt/1  "dwm_dt"

== system MotorControlSim_OpenLoopPWM/PMSM1/Park transform ==
  theta_e : Inport
  "ualpha, ubeta" : Inport  Port=2
  Demux : Demux  Outputs=2
  Gain : Gain  Gain=-1
  Matrix Concatenate : Concatenate  Mode=Multidimensional array  ConcatenateDimension=2
  Matrix Concatenate1 : Concatenate  Mode=Multidimensional array  ConcatenateDimension=2
  Matrix Concatenate2 : Concatenate  Mode=Multidimensional array
  Product1 : Product  Multiplication=Matrix(*)
  Sin : Trigonometry  Operator=cos
  Sin1 : Trigonometry
  ud : Outport
  uq : Outport  Port=2
  wires:
  Demux/2 -> uq/1  "uq"
  Product1/1 -> Demux/1  "ud, uq"
  Gain/1 -> Matrix Concatenate1/1
  Matrix Concatenate1/1 -> Matrix Concatenate2/2
  Sin1/1 -> Gain/1, Matrix Concatenate/2
  Matrix Concatenate2/1 -> Product1/1
  Matrix Concatenate/1 -> Matrix Concatenate2/1
  Sin/1 -> Matrix Concatenate/1, Matrix Concatenate1/2
  theta_e/1 -> Sin1/1, Sin/1
  Demux/1 -> ud/1  "ud"
  "ualpha, ubeta"/1 -> Product1/2

== system MotorControlSim_OpenLoopPWM/PMSM1/Phase voltage calculation ==
  ua0 : Inport
  ub0 : Inport  Port=2
  uc0 : Inport  Port=3
  Add : Sum  Inputs=+++
  Gain : Gain  Gain=1/3
  Subtract : Sum  Inputs=+-
  Subtract1 : Sum  Inputs=+-
  Subtract2 : Sum  Inputs=+-
  ua : Outport
  ub : Outport  Port=2
  uc : Outport  Port=3
  wires:
  uc0/1 -> Add/3, Subtract2/1
  Subtract2/1 -> uc/1
  Subtract/1 -> ua/1
  Gain/1 -> Subtract/2, Subtract1/2, Subtract2/2  "un"
  Add/1 -> Gain/1
  ua0/1 -> Subtract/1, Add/1
  ub0/1 -> Add/2, Subtract1/1
  Subtract1/1 -> ub/1

== system MotorControlSim_OpenLoopPWM/PMSM2/Clarke transform ==
  ua : Inport
  ub : Inport  Port=2
  uc : Inport  Port=3
  Constant : Constant  Value=[1 -1/2 -1/2; 0 sqrt(3)/2 -sqrt(3)/2]
  Gain2 : Gain  Gain=2/3
  Mux : Mux  Inputs=3
  Product : Product  Multiplication=Matrix(*)
  "ualpha, ubeta" : Outport
  wires:
  Gain2/1 -> Product/1
  ub/1 -> Mux/2
  Constant/1 -> Gain2/1
  Mux/1 -> Product/2
  Product/1 -> "ualpha, ubeta"/1
  uc/1 -> Mux/3
  ua/1 -> Mux/1

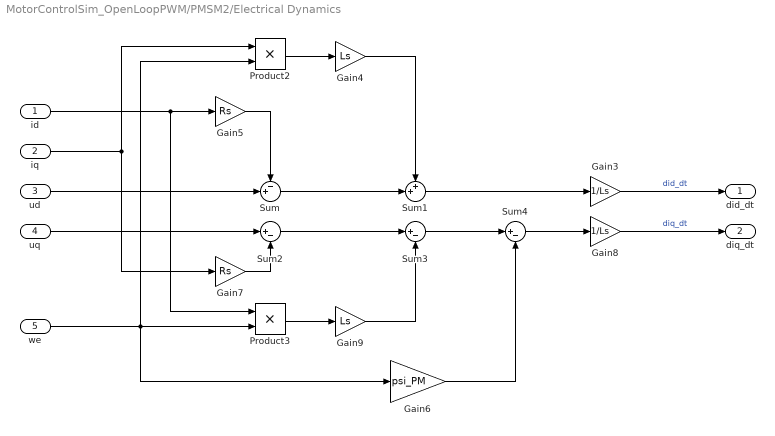
== system MotorControlSim_OpenLoopPWM/PMSM2/Electrical Dynamics ==
  id : Inport
  iq : Inport  Port=2
  ud : Inport  Port=3
  uq : Inport  Port=4
  we : Inport  Port=5
  Gain3 : Gain  Gain=1/Ls
  Gain4 : Gain  Gain=Ls
  Gain5 : Gain  Gain=Rs
  Gain6 : Gain  Gain=psi_PM
  Gain7 : Gain  Gain=Rs
  Gain8 : Gain  Gain=1/Ls
  Gain9 : Gain  Gain=Ls
  Product2 : Product
  Product3 : Product
  Sum : Sum  Inputs=-+|
  Sum1 : Sum  Inputs=++|
  Sum2 : Sum  Inputs=|+-
  Sum3 : Sum  Inputs=|+-
  Sum4 : Sum  Inputs=|+-
  did_dt : Outport
  diq_dt : Outport  Port=2
  wires:
  Product2/1 -> Gain4/1
  Gain9/1 -> Sum3/2
  Gain7/1 -> Sum2/2
  Sum/1 -> Sum1/2
  iq/1 -> Gain7/1, Product2/1
  Product3/1 -> Gain9/1
  Sum4/1 -> Gain8/1
  ud/1 -> Sum/2
  Gain4/1 -> Sum1/1
  Gain6/1 -> Sum4/2
  Gain8/1 -> diq_dt/1  "diq_dt"
  Gain5/1 -> Sum/1
  id/1 -> Product3/1, Gain5/1
  uq/1 -> Sum2/1
  we/1 -> Product2/2, Gain6/1, Product3/2
  Sum3/1 -> Sum4/1
  Sum1/1 -> Gain3/1
  Gain3/1 -> did_dt/1  "did_dt"
  Sum2/1 -> Sum3/1

== system MotorControlSim_OpenLoopPWM/PMSM2/Inverse Clarke ==
  "ialpha, ibeta" : Inport
  Constant1 : Constant  Value=[1 0; -1/2 sqrt(3)/2; -1/2 -sqrt(3)/2]
  Demux1 : Demux  Outputs=3
  Matrix Multiply : Product  Multiplication=Matrix(*)
  ia : Outport
  ib : Outport  Port=2
  ic : Outport  Port=3
  wires:
  Matrix Multiply/1 -> Demux1/1
  Constant1/1 -> Matrix Multiply/1
  Demux1/2 -> ib/1  "ib"
  Demux1/3 -> ic/1  "ic"
  Demux1/1 -> ia/1  "ia"
  "ialpha, ibeta"/1 -> Matrix Multiply/2

== system MotorControlSim_OpenLoopPWM/PMSM2/Inverse Park ==
  theta_e : Inport
  id : Inport  Port=2
  iq : Inport  Port=3
  Cos : Trigonometry  Operator=cos
  Gain3 : Gain  Gain=-1
  Matrix Concatenate3 : Concatenate  Mode=Multidimensional array  ConcatenateDimension=2
  Matrix Concatenate4 : Concatenate  Mode=Multidimensional array  ConcatenateDimension=2
  Matrix Concatenate5 : Concatenate  Mode=Multidimensional array
  Mux1 : Mux  Inputs=2
  Product2 : Product  Multiplication=Matrix(*)
  Sin2 : Trigonometry
  "ialpha, ibeta" : Outport
  wires:
  theta_e/1 -> Sin2/1, Cos/1
  Gain3/1 -> Matrix Concatenate3/2
  Cos/1 -> Matrix Concatenate3/1, Matrix Concatenate4/2
  Mux1/1 -> Product2/2
  iq/1 -> Mux1/2
  Matrix Concatenate4/1 -> Matrix Concatenate5/2
  Matrix Concatenate5/1 -> Product2/1
  Product2/1 -> "ialpha, ibeta"/1  "ialpha, ibeta"
  Sin2/1 -> Matrix Concatenate4/1, Gain3/1
  Matrix Concatenate3/1 -> Matrix Concatenate5/1
  id/1 -> Mux1/1

== system MotorControlSim_OpenLoopPWM/PMSM2/Mechanical dynamics ==
  Te : Inport
  TL : Inport  Port=2
  wm : Inport  Port=3
  Gain7 : Gain  Gain=1/J
  Gain9 : Gain  Gain=B
  Sum5 : Sum  Inputs=|+-
  Sum6 : Sum  Inputs=|+-
  dwm_dt : Outport
  wires:
  Gain9/1 -> Sum6/2
  TL/1 -> Sum5/2
  Te/1 -> Sum5/1
  Sum6/1 -> Gain7/1
  wm/1 -> Gain9/1
  Sum5/1 -> Sum6/1
  Gain7/1 -> dwm_dt/1  "dwm_dt"
